simulink model "untitled6"  (R2024b)
settings: Solver=VariableStepAuto  StartTime=0.0  StopTime=10.0  RelTol=1e-3
undefined symbols (not defined in the file or in its folder): DiscIntNeverNeededParam
libraries: simulink x4
(part 2 of 2)

== system untitled6/Wheel Dynamics/Wrr Subsystem ==
  Trr : Inport
  Frr : Inport  Port=2
  -1/b3 : Gain  Gain=-1/0.1
  Discrete Derivative : simulink/Discrete/Discrete Derivative  gainval=1.0  ICPrevScaledInput=0.0  OutMin=[]  OutMax=[]  OutDataType=fixdt(1, 16)  OutScaling=2^-10  DoSatur=off
  Iw3 : Constant  Value=2.5
  Product5 : Product
  Product6 : Product
  Rw3 : Constant  Value=0.228
  Sum3 : Sum  Inputs=|++-
  Wrr : Outport
  wires:
  Sum3/1 -> -1/b3/1
  Product5/1 -> Sum3/1
  Frr/1 -> Product5/2
  -1/b3/1 -> Discrete Derivative/1, Wrr/1
  Iw3/1 -> Product6/1
  Product6/1 -> Sum3/2
  Trr/1 -> Sum3/3
  Discrete Derivative/1 -> Product6/2
  Rw3/1 -> Product5/1

== system untitled6/Side slip angle/Vel of whee due to veh speedl/Subsystem ==
  Vy : Inport
  Vx : Inport  Port=2
  Rf : Inport  Port=3
  Yaw rate : Inport  Port=4
  Comp1 : Inport  Port=5
  Comp2 : Inport  Port=6
  Math Function : Math  Operator=square
  Math Function1 : Math  Operator=square
  Product : Product  Inputs=3
  Product1 : Product  Inputs=3
  Sqrt1 : Sqrt
  Subtract : Sum  Inputs=+-
  Subtract1 : Sum
  Subtract2 : Sum
  VBfl : Outport
  wires:
  Yaw rate/1 -> Product/2, Product1/2
  Subtract1/1 -> Sqrt1/1
  Math Function1/1 -> Subtract1/2
  Subtract/1 -> Math Function/1
  Product1/1 -> Subtract2/2
  Rf/1 -> Product1/1, Product/1
  Sqrt1/1 -> VBfl/1
  Subtract2/1 -> Math Function1/1
  Math Function/1 -> Subtract1/1
  Product/1 -> Subtract/2
  Vx/1 -> Subtract/1
  Vy/1 -> Subtract2/1
  Comp2/1 -> Product1/3
  Comp1/1 -> Product/3

== system untitled6/Side slip angle/Vel of whee due to veh speedl/Subsystem1 ==
  Vy : Inport
  Vx : Inport  Port=2
  Rf : Inport  Port=3
  Yaw rate : Inport  Port=4
  Comp1 : Inport  Port=5
  Comp2 : Inport  Port=6
  Math Function : Math  Operator=square
  Math Function1 : Math  Operator=square
  Product : Product  Inputs=3
  Product1 : Product  Inputs=3
  Sqrt1 : Sqrt
  Subtract : Sum
  Subtract1 : Sum
  Subtract2 : Sum
  VBfr : Outport
  wires:
  Comp1/1 -> Product/3
  Comp2/1 -> Product1/3
  Vy/1 -> Subtract2/1
  Vx/1 -> Subtract/1
  Product/1 -> Subtract/2
  Math Function/1 -> Subtract1/1
  Subtract2/1 -> Math Function1/1
  Sqrt1/1 -> VBfr/1
  Rf/1 -> Product/1, Product1/1
  Product1/1 -> Subtract2/2
  Subtract/1 -> Math Function/1
  Math Function1/1 -> Subtract1/2
  Subtract1/1 -> Sqrt1/1
  Yaw rate/1 -> Product1/2, Product/2

== system untitled6/Side slip angle/Vel of whee due to veh speedl/Subsystem2 ==
  Vy : Inport
  Vx : Inport  Port=2
  Rl : Inport  Port=3
  Yaw rate : Inport  Port=4
  Comp1 : Inport  Port=5
  Comp2 : Inport  Port=6
  Math Function : Math  Operator=square
  Math Function1 : Math  Operator=square
  Product : Product  Inputs=3
  Product1 : Product  Inputs=3
  Sqrt1 : Sqrt
  Subtract : Sum  Inputs=+-
  Subtract1 : Sum
  Subtract2 : Sum
  VBrl : Outport
  wires:
  Yaw rate/1 -> Product/2, Product1/2
  Subtract1/1 -> Sqrt1/1
  Math Function1/1 -> Subtract1/2
  Subtract/1 -> Math Function/1
  Product1/1 -> Subtract2/2
  Rl/1 -> Product1/1, Product/1
  Sqrt1/1 -> VBrl/1
  Subtract2/1 -> Math Function1/1
  Math Function/1 -> Subtract1/1
  Product/1 -> Subtract/2
  Vx/1 -> Subtract/1
  Vy/1 -> Subtract2/1
  Comp2/1 -> Product1/3
  Comp1/1 -> Product/3

== system untitled6/Side slip angle/Vel of whee due to veh speedl/Subsystem3 ==
  Vy : Inport
  Vx : Inport  Port=2
  Rl : Inport  Port=3
  Yaw rate : Inport  Port=4
  Comp1 : Inport  Port=5
  Comp2 : Inport  Port=6
  Math Function : Math  Operator=square
  Math Function1 : Math  Operator=square
  Product : Product  Inputs=3
  Product1 : Product  Inputs=3
  Sqrt1 : Sqrt
  Subtract : Sum
  Subtract1 : Sum
  Subtract2 : Sum  Inputs=+-
  VBrr : Outport
  wires:
  Comp1/1 -> Product/3
  Comp2/1 -> Product1/3
  Vy/1 -> Subtract2/1
  Vx/1 -> Subtract/1
  Product/1 -> Subtract/2
  Math Function/1 -> Subtract1/1
  Subtract2/1 -> Math Function1/1
  Sqrt1/1 -> VBrr/1
  Rl/1 -> Product/1, Product1/1
  Product1/1 -> Subtract2/2
  Subtract/1 -> Math Function/1
  Math Function1/1 -> Subtract1/2
  Subtract1/1 -> Sqrt1/1
  Yaw rate/1 -> Product1/2, Product/2

== system untitled6/Tire model/Subsystem1/Subsystem ==
  In1 : Inport
  C1 : Constant  Value=1.280
  C2 : Constant  Value=23.99
  C3 : Constant  Value=0.52
  Constant : Constant
  Gain : Gain  Gain=-1
  Math Function : Math
  Product : Product
  Product1 : Product
  Product2 : Product
  Subtract : Sum  Inputs=+-
  Subtract1 : Sum  Inputs=+-
  UrSfl : Outport
  wires:
  C2/1 -> Gain/1
  Gain/1 -> Product/1
  C3/1 -> Product2/1
  C1/1 -> Product1/2
  Product2/1 -> Subtract1/2
  Constant/1 -> Subtract/1
  Product/1 -> Math Function/1
  Math Function/1 -> Subtract/2
  Subtract/1 -> Product1/1
  Product1/1 -> Subtract1/1
  In1/1 -> Product2/2, Product/2
  Subtract1/1 -> UrSfl/1

== system untitled6/Tire model/Subsystem2/Subsystem ==
  In1 : Inport
  C1 : Constant  Value=1.280
  C2 : Constant  Value=23.99
  C3 : Constant  Value=0.52
  Constant : Constant
  Gain : Gain  Gain=-1
  Math Function : Math
  Product : Product
  Product1 : Product
  Product2 : Product
  Subtract : Sum  Inputs=+-
  Subtract1 : Sum  Inputs=+-
  UrSfl : Outport
  wires:
  Subtract1/1 -> UrSfl/1
  In1/1 -> Product/2, Product2/2
  Product1/1 -> Subtract1/1
  Subtract/1 -> Product1/1
  Math Function/1 -> Subtract/2
  Product/1 -> Math Function/1
  Constant/1 -> Subtract/1
  Product2/1 -> Subtract1/2
  C1/1 -> Product1/2
  C3/1 -> Product2/1
  Gain/1 -> Product/1
  C2/1 -> Gain/1

== system untitled6/Tire model/Subsystem3/Subsystem ==
  In1 : Inport
  C1 : Constant  Value=1.280
  C2 : Constant  Value=23.99
  C3 : Constant  Value=0.52
  Constant : Constant
  Gain : Gain  Gain=-1
  Math Function : Math
  Product : Product
  Product1 : Product
  Product2 : Product
  Subtract : Sum  Inputs=+-
  Subtract1 : Sum  Inputs=+-
  UrSfl : Outport
  wires:
  C2/1 -> Gain/1
  Gain/1 -> Product/1
  C3/1 -> Product2/1
  C1/1 -> Product1/2
  Product2/1 -> Subtract1/2
  Constant/1 -> Subtract/1
  Product/1 -> Math Function/1
  Math Function/1 -> Subtract/2
  Subtract/1 -> Product1/1
  Product1/1 -> Subtract1/1
  In1/1 -> Product2/2, Product/2
  Subtract1/1 -> UrSfl/1

== system untitled6/Tire model/Subsystem4/Subsystem ==
  In1 : Inport
  C1 : Constant  Value=1.280
  C2 : Constant  Value=23.99
  C3 : Constant  Value=0.52
  Constant : Constant
  Gain : Gain  Gain=-1
  Math Function : Math
  Product : Product
  Product1 : Product
  Product2 : Product
  Subtract : Sum  Inputs=+-
  Subtract1 : Sum  Inputs=+-
  UrSfl : Outport
  wires:
  Subtract1/1 -> UrSfl/1
  In1/1 -> Product/2, Product2/2
  Product1/1 -> Subtract1/1
  Subtract/1 -> Product1/1
  Math Function/1 -> Subtract/2
  Product/1 -> Math Function/1
  Constant/1 -> Subtract/1
  Product2/1 -> Subtract1/2
  C1/1 -> Product1/2
  C3/1 -> Product2/1
  Gain/1 -> Product/1
  C2/1 -> Gain/1

== system untitled6/Vertical load /Vertical Fores/Vertical force fl ==
  g : Inport
  lf : Inport  Port=2
  l : Inport  Port=3
  ax : Inport  Port=4
  m : Inport  Port=5
  Hcg : Inport  Port=6
  tf : Inport  Port=7
  ay : Inport  Port=8
  Constant : Constant  Value=0.5
  Divide : Product  Inputs=*/
  Divide1 : Product  Inputs=*/
  Divide2 : Product  Inputs=*/
  Product{,1..3} (4 alike) : Product
  Product4 : Product  Inputs=3
  Subtract : Sum  Inputs=+-
  Subtract1 : Sum  Inputs=+-
  Fz,fl : Outport
  wires:
  Product2/1 -> Subtract1/2
  Product/1 -> Subtract/1
  g/1 -> Product3/1, Product/1
  Hcg/1 -> Divide2/1, Divide1/1
  Subtract1/1 -> Product4/3
  Product4/1 -> Fz,fl/1
  l/1 -> Divide/2, Divide1/2
  m/1 -> Product4/2
  Divide1/1 -> Product1/2
  Divide/1 -> Product/2
  ay/1 -> Product2/2
  Product3/1 -> Divide2/2
  Subtract/1 -> Product4/1
  Divide2/1 -> Product2/1
  Product1/1 -> Subtract/2
  ax/1 -> Product1/1
  Constant/1 -> Subtract1/1
  lf/1 -> Divide/1
  tf/1 -> Product3/2

== system untitled6/Vertical load /Vertical Fores/Vertical force fr ==
  g : Inport
  lf : Inport  Port=2
  l : Inport  Port=3
  ax : Inport  Port=4
  m : Inport  Port=5
  tf : Inport  Port=6
  ay : Inport  Port=7
  Hcg : Inport  Port=8
  Constant : Constant  Value=0.5
  Divide : Product  Inputs=*/
  Divide1 : Product  Inputs=*/
  Divide2 : Product  Inputs=*/
  Product{,1..3} (4 alike) : Product
  Product4 : Product  Inputs=3
  Subtract : Sum  Inputs=+-
  Subtract1 : Sum
  Fz,fr : Outport
  wires:
  tf/1 -> Product3/2
  lf/1 -> Divide/1
  Constant/1 -> Subtract1/1
  ax/1 -> Product1/1
  Product1/1 -> Subtract/2
  Divide2/1 -> Product2/1
  Subtract/1 -> Product4/1
  Product3/1 -> Divide2/2
  ay/1 -> Product2/2
  Divide/1 -> Product/2
  Divide1/1 -> Product1/2
  m/1 -> Product4/2
  l/1 -> Divide1/2, Divide/2
  Product4/1 -> Fz,fr/1
  Subtract1/1 -> Product4/3
  Hcg/1 -> Divide1/1, Divide2/1
  g/1 -> Product/1, Product3/1
  Product/1 -> Subtract/1
  Product2/1 -> Subtract1/2

== system untitled6/Vertical load /Vertical Fores/Vertical force rl ==
  g : Inport
  lr : Inport  Port=2
  l : Inport  Port=3
  ax : Inport  Port=4
  m : Inport  Port=5
  Hcg : Inport  Port=6
  tr : Inport  Port=7
  ay : Inport  Port=8
  Constant : Constant  Value=0.5
  Divide : Product  Inputs=*/
  Divide1 : Product  Inputs=*/
  Divide2 : Product  Inputs=*/
  Product{,1..3} (4 alike) : Product
  Product4 : Product  Inputs=3
  Subtract : Sum
  Subtract1 : Sum  Inputs=+-
  Fz,rl : Outport
  wires:
  tr/1 -> Product3/2
  lr/1 -> Divide/1
  Constant/1 -> Subtract1/1
  ax/1 -> Product1/1
  Product1/1 -> Subtract/2
  Divide2/1 -> Product2/1
  Subtract/1 -> Product4/1
  Product3/1 -> Divide2/2
  ay/1 -> Product2/2
  Divide/1 -> Product/2
  Divide1/1 -> Product1/2
  m/1 -> Product4/2
  l/1 -> Divide1/2, Divide/2
  Product4/1 -> Fz,rl/1
  Subtract1/1 -> Product4/3
  Hcg/1 -> Divide1/1, Divide2/1
  g/1 -> Product/1, Product3/1
  Product/1 -> Subtract/1
  Product2/1 -> Subtract1/2

== system untitled6/Vertical load /Vertical Fores/Vertical force rr ==
  g : Inport
  lr : Inport  Port=2
  l : Inport  Port=3
  ax : Inport  Port=4
  m : Inport  Port=5
  Hcg : Inport  Port=6
  tr : Inport  Port=7
  ay : Inport  Port=8
  Constant : Constant  Value=0.5
  Divide : Product  Inputs=*/
  Divide1 : Product  Inputs=*/
  Divide2 : Product  Inputs=*/
  Product{,1..3} (4 alike) : Product
  Product4 : Product  Inputs=3
  Subtract : Sum
  Subtract1 : Sum
  Fz,rr : Outport
  wires:
  Product2/1 -> Subtract1/2
  Product/1 -> Subtract/1
  g/1 -> Product3/1, Product/1
  Hcg/1 -> Divide2/1, Divide1/1
  Subtract1/1 -> Product4/3
  Product4/1 -> Fz,rr/1
  l/1 -> Divide/2, Divide1/2
  m/1 -> Product4/2
  Divide1/1 -> Product1/2
  Divide/1 -> Product/2
  ay/1 -> Product2/2
  Product3/1 -> Divide2/2
  Subtract/1 -> Product4/1
  Divide2/1 -> Product2/1
  Product1/1 -> Subtract/2
  ax/1 -> Product1/1
  Constant/1 -> Subtract1/1
  lr/1 -> Divide/1
  tr/1 -> Product3/2
